simulink model "stateflow1"  (R2015a)
settings: Solver=ode3  StartTime=0.0  StopTime=30  RelTol=1e-3
undefined symbols (not defined in the file or in its folder): sigbuilder_block
libraries: legoev3lib x2
settings Model: SimulationMode=external  ExtModeTrigDuration=2  Creator=Keshav  LastModifiedBy=Keshav
settings OptimizationCC: OptimizeModelRefInitCode=on  LifeSpan=1
settings DebuggingCC: UnderspecifiedInitializationDetection=Classic  MergeDetectMultiDrivingBlocksExec=none
settings HardwareCC: ProdLargestAtomicInteger=Long  ProdLargestAtomicFloat=Float  ProdEndianess=LittleEndian  ProdHWDeviceType=ARM Compatible->ARM 9
settings RTWCC: SystemTargetFile=realtime.tlc  GenerateMakefile=off  TemplateMakefile=realtime.tmf  Description=Run on Target Hardware  RTWVerbose=off
settings ERTTargetCC: CombineOutputUpdateFcns=off  ExtModeMexArgs=0 1 9600  ERTSrcFileBannerTemplate=realtime_code_template.cgt  ERTHdrFileBannerTemplate=realtime_code_template.cgt  ERTDataSrcFileTemplate=realtime_code_template.cgt  ERTDataHdrFileTemplate=realtime_code_template.cgt  ERTCustomFileTemplate=realtime_file_process.tlc

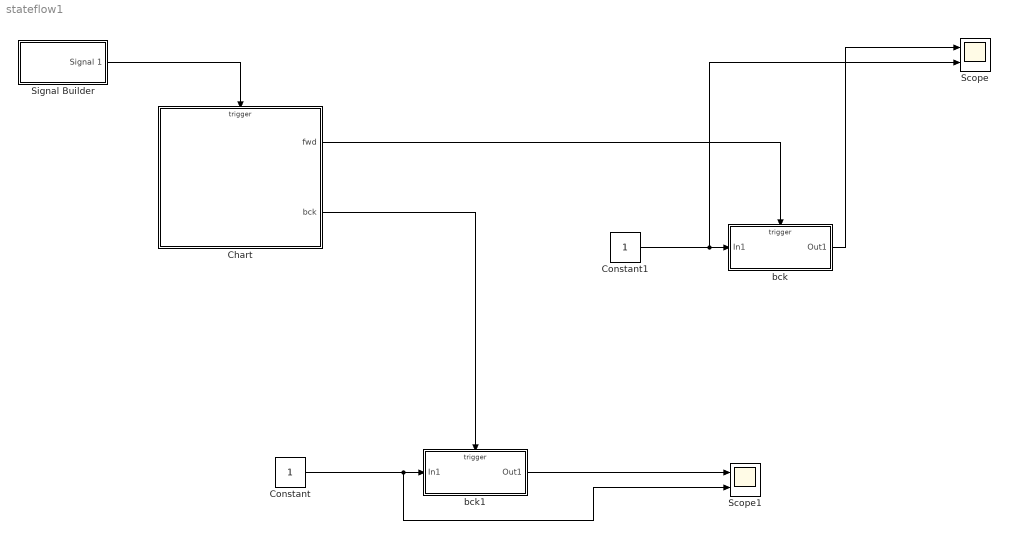
== system stateflow1 ==
  Chart : Stateflow chart  TreatAsAtomicUnit=on
  Constant : Constant
  Constant1 : Constant
  Scope : Scope  NumInputPorts=2
      settings: YMin=-1~-30  YMax=1~-30
  Scope1 : Scope  NumInputPorts=2
      settings: YMin=-5~-5  YMax=5~5
  Signal Builder : Subsystem  Tag=STV Subsys  LoadFcn=sigbuilder_block('load');  StartFcn=sigbuilder_block('start');  StopFcn=sigbuilder_block('stop');  ClipboardFcn=sigbuilder_block('clipboard');  mask(Sigbuilder block){}
      mask help: Simulink:masks:SigbuilderBlock_MD
      mask init:
      | if ~strcmp(get_param(bdroot(gcbh),'SimulationStatus'),'stopped') tuvar = sigbuilder_block('maskInit'); end
      settings: CopyFcn=sigbuilder_block('copy');  DeleteFcn=sigbuilder_block('delete');  ModelCloseFcn=sigbuilder_block('modelClose');  PreSaveFcn=sigbuilder_block('preSave');  PauseFcn=sigbuilder_block('pause');  ContinueFcn=sigbuilder_block('continue');  NameChangeFcn=sigbuilder_block('namechange');  OpenFcn=sigbuilder_block('open',[437.6 199.2 550.4 400 ]);  CloseFcn=sigbuilder_block('close');
      mask Display: plot(0, 0, 100, 100,[2, 2, 32, 32, 2], [68, 8, 8, 68, 68],[32, 2], [38, 38], [32, 19, 2],[53, 60, 44], [32, 17, 17, 2],[16, 16, 31, 31]);txt = getActiveGroup(gcbh);text(2, 100, txt,'verticalAlignment', 'top');
  bck : Subsystem  TreatAsAtomicUnit=on
  bck1 : Subsystem  TreatAsAtomicUnit=on
  wires:
  Constant1/1 -> Scope/2, bck/1(In1)
  Signal Builder/1(Signal 1) -> Chart/Trigger
  Chart/1(fwd) -> bck/Trigger
  Constant/1 -> Scope1/2, bck1/1(In1)
  Chart/2(bck) -> bck1/Trigger
  bck/1(Out1) -> Scope/1
  bck1/1(Out1) -> Scope1/1

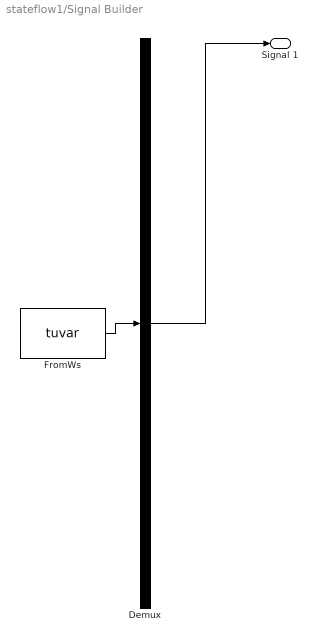
== system stateflow1/Signal Builder ==
  Demux : Demux  Tag=STV Demux  Outputs=1
  FromWs : FromWorkspace  Tag=STV FromWs  VariableName=tuvar  SampleTime=0
      SigBuilderData=|
      | common.afterFinalStr = 'Extrapolate'
      | common.sampleTime = 0
      | dataSet.timeRange = [0 10]
      | dataSet.name = 'Group 1'
      | sbobj.Groups.Name = 'Group 1'
      | sbobj.Groups.Signals.Name = 'Signal 1'
      | sbobj.Groups.Signals.XData = [0 10]
      | sbobj.Groups.Signals.YData = [1 1]
  Signal 1 : Outport  Tag=STV Outport
  wires:
  Demux/1 -> Signal 1/1
  FromWs/1 -> Demux/1

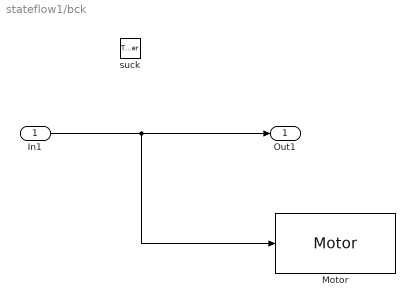
== system stateflow1/bck ==
  In1 : Inport
  suck : TriggerPort
  Motor : legoev3lib/Motor  sportNumber=A  sstopAction=Brake
  Out1 : Outport
  wires:
  In1/1 -> Motor/1, Out1/1

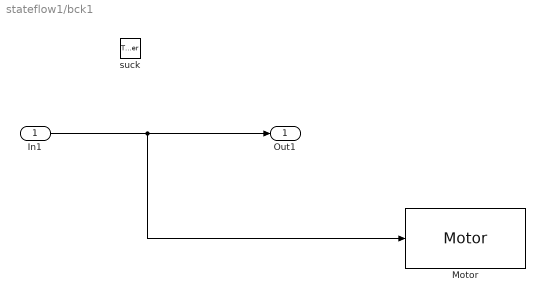
== system stateflow1/bck1 ==
  In1 : Inport
  suck : TriggerPort
  Motor : legoev3lib/Motor  sportNumber=A  sstopAction=Brake
  Out1 : Outport
  wires:
  In1/1 -> Motor/1, Out1/1

== stateflow chart stateflow1/Chart ==
  note: ?
  state mtr_fwd
    du:fwd = 1;
  state mtr_bck
    du:bck=1;
  (default) -> mtr_fwd : entry
  mtr_fwd -> mtr_bck : after(5, sec)
  mtr_bck -> mtr_fwd : after(5, sec)
  events: fwd output EITHER_EDGE_EVENT; bck output EITHER_EDGE_EVENT; entry input RISING_EDGE_EVENT
